simulink model "flightControlSystem"  (R2024b)
settings: Solver=ode3  StartTime=0  StopTime=TFinal  FixedStep=Ts  RelTol=1e-3  EnableMultiTasking=on
undefined symbols (not defined in the file): codertarget, Controller, DiscIntNeverNeededParam, Discrete, Estimator, g, gray, init, orient_ref, pos_ref, Rec, SDTV, Sensors, strel, Time, Ts, var_acc_angle_N, var_bias_gyr_N, var_gyro_p_N, Vehicle
libraries: simulink x51, matrix_library x8, slpidlib x4, ctrlSharedLib x4, sharedtransform x3, visionconversions x2, visionmorphops x2, parrotlib x1
(part 3 of 3)

== system flightControlSystem/Control System/State Estimator/XY Position Estimator/EstimatorVelocity/xy velocity w//o angular velocity compensation ==
  note: Optical flow raw readings are converted to velocity in m/s based on the estimated altitude
  optical_flow : Inport
  z_estimate : Inport  Port=2
  " " : Product  Inputs=**
  Compare To Constant : simulink/Logic and Bit Operations/Compare To Constant  relop=<  const=200*4  OutDataTypeStr=boolean
  Counter Free-Running : simulink/Sources/Counter Free-Running  NumBits=32  tsamp=-1
  Gain : Gain  Gain=-1
  Select dxy : Selector  InputPortWidth=3  IndexOptions=Index vector (dialog)  Indices=[1 2]  OutputSizes=1
  Switch : Switch  Criteria=u2 > Threshold  SaturateOnIntegerOverflow=off  InputSameDT=off
  opticalFlowErrorCorrect : Gain  Gain=1.15
  optical_flow_dx_dy : Outport
  wires:
  Select dxy/1 -> optical_flow_dx_dy/1  "optical_flow_dx_dy"
  " "/1 -> opticalFlowErrorCorrect/1
  opticalFlowErrorCorrect/1 -> Switch/3
  Gain/1 -> " "/2
  Switch/1 -> Select dxy/1
  Counter Free-Running/1 -> Compare To Constant/1
  Compare To Constant/1 -> Switch/2
  optical_flow/1 -> " "/1, Switch/1
  z_estimate/1 -> Gain/1

== stateflow chart flightControlSystem/Control System/Path Planning/Line-follower Algorithm ==
  state Land
    entry:
    x0 = x0;
    y0 = y0;
    z0 = 0;
    yaw0 = yaw0;
  state Dock
    during:
    x0 = x0;
    y0 = y0;
    z0 = z0 + 0.001;
    yaw0 = yaw0;
  state Position
    during:
    x0 = x0 + cos(yaw0)*0.0001;
    y0 = y0 + sin(yaw0)*0.0001;
    z0 = z0;
    yaw0 = yaw0;
  state Left_Turn
    during:
    x0 = x0;
    y0 = y0;
    z0 = z0;
    yaw0 = yaw0 - 0.001;
  state Takeoff
    entry:
    x0 = 0;
    y0 = 0;
    z0 = -1.1;
    yaw0 = 0;
  state Hover
    during:
    x0 = x0;
    y0 = y0;
    z0 = z0;
    yaw0 = yaw0;
  state Move
    during:
    x0 = x0 + cos(yaw0)*0.001;
    y0 = y0 + sin(yaw0)*0.001;
    z0 = z0;
    yaw0 = yaw0;
  state Right_Turn
    during:
    x0 = x0;
    y0 = y0;
    z0 = z0;
    yaw0 = yaw0 + 0.001;
  note: <- Forward == 0?
  note: turn: Detects path forward based solely on positive pixel value in middle front. Ignores alignment.
      | forward: Requires both positive pixel value in middle front and correct alignment for path detection.
      | RL: Used to choose a direction when both Right and Left are detected
      | tcorrection: similar to rcorrection except its scope is in middle row
      | r/lcorrection: counts no. of pixels from left and right to middle and correct alignment
  state Left_Correction
    during:
    x0 = x0;
    y0 = y0;
    z0 = z0;
    yaw0 = yaw0 + 0.0005;
  state Right_Correction
    during:
    x0 = x0;
    y0 = y0;
    z0 = z0;
    yaw0 = yaw0 - 0.0005;
  Right_Correction -> Left_Turn [order 4] : [turn == 0 & Left == 1 & RL < 0]
  Position -> Dock : [dock == 1]
  Dock -> Land : [z0 >= -0.1]
  Left_Correction -> Left_Turn [order 3] : [turn == 0 & Left == 1 & RL < 0]
  Hover -> Left_Turn [order 2] : [turn == 0 & Left == 1]
  Move -> Position [order 5] : [turn == 0 & Right == 0 & Left == 0]
  Left_Turn -> Move : [Forward == 1]
  Move -> Left_Turn [order 2] : [turn == 0 & Left == 1 & RL < 0]
  Hover -> Right_Turn [order 3] : [turn == 0 & Right == 1]
  (default) -> Takeoff
  Move -> Right_Turn [order 1] : [turn == 0 & Right == 1 & RL > 0]
  Takeoff -> Hover : after(4,sec)
  Hover -> Move [order 1] : [Forward == 1]
  Right_Turn -> Move : [Forward == 1]
  Left_Correction -> Right_Turn [order 4] : [turn == 0 & Right == 1 & RL > 0]
  Hover -> Right_Correction [order 5] : [tcorrection > 0]
  Hover -> Left_Correction [order 4] : [tcorrection < 0]
  Move -> Left_Correction [order 4] : [Forward == 0 & rcorrection < lcorrection]
  Left_Correction -> Move [order 1] : [Forward == 1]
  Move -> Right_Correction [order 3] : [Forward == 0 & rcorrection > lcorrection]
  Right_Correction -> Move [order 1] : [Forward == 1]
  Right_Correction -> Right_Turn [order 3] : [turn == 0 & Right == 1 & RL > 0]
  Left_Correction -> Right_Correction [order 2] : [rcorrection > lcorrection]
  Right_Correction -> Left_Correction [order 2] : [rcorrection < lcorrection]
  data: yaw0 output; x0 output; Forward input; y0 output; z0 output; Right input; rcorrection input; turn input; lcorrection input; Left input; dock input; tcorrection input; RL input

== matlab function flightControlSystem/Control System/Controller/Position Controller/Position error transformation (Earth to Body frame) ==
  data: yaw input; xy_err_earth input; xy_err_body output
function xy_err_body = fcn(yaw,xy_err_earth)

transformation = [cos(yaw), sin(yaw); -sin(yaw),  cos(yaw)];
xy_err_body = transformation * xy_err_earth;


end
